simulink library "threeTetherThreeSurfaceCtrl_cl"  (R2022a)
settings: Solver=VariableStepAuto  StartTime=0.0  StopTime=10.0  RelTol=1e-3
undefined symbols (not defined in the file or in its folder): altitudeCtrlShutOffDelay, expOffset, filteredPIDController, filteredPIDController_ul, FLIGHTCONTROLLER, fltCtrl, initialDelay, initializeBussesFromBlock
settings Model: Creator=mcobb  LastModifiedBy=lhill8
settings SolverCC: AlgebraicLoopSolver=TrustRegion
settings DebuggingCC: UnconnectedInputMsg=warning  UnconnectedOutputMsg=warning  UnconnectedLineMsg=warning  SFMachineParentedDataDiag=warning  ArithmeticOperatorsInVariantConditions=warning
settings SFSimCC: CustomCodeUndefinedFunction=UseInterfaceOnly

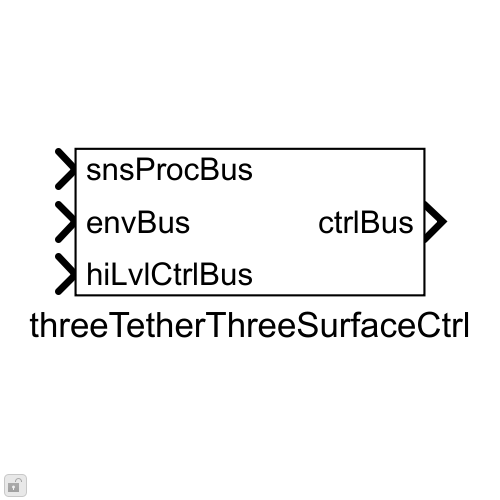
[thumbnail: Simulink's stored preview of the top-level diagram]
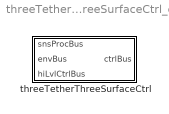
== system threeTetherThreeSurfaceCtrl_cl ==
  threeTetherThreeSurfaceCtrl : Subsystem  LoadFcn=initializeBussesFromBlock(gcb)  InitFcn=initializeBussesFromBlock(gcb)  StartFcn=initializeBussesFromBlock(gcb)  VariantControl=strcmpi(FLIGHTCONTROLLER,'threeTetherThreeSurfaceCtrl')  mask{ctrl=fltCtrl}
      mask prompts: ctrl "Controller Object"

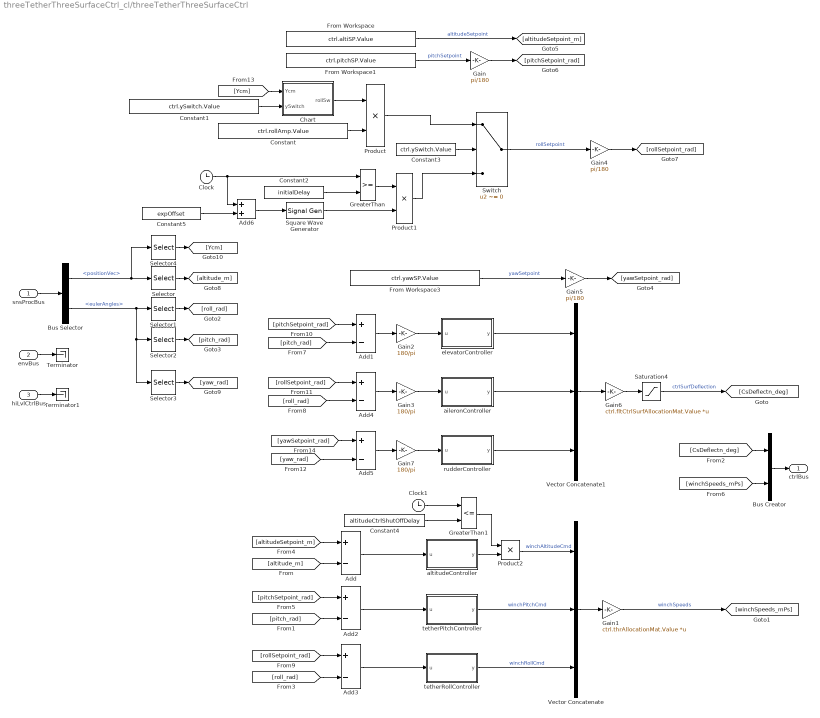
== system threeTetherThreeSurfaceCtrl_cl/threeTetherThreeSurfaceCtrl ==
  snsProcBus : Inport  OutDataTypeStr=Bus: sensorsProcessingBus
  envBus : Inport  Port=2  OutDataTypeStr=Bus: envBus
  hiLvlCtrlBus : Inport  Port=3  OutDataTypeStr=Bus: hiLvlCtrlBus
  Add{,1..5} (6 alike) : Sum  Inputs=+-
  Add6 : Sum
  Bus Creator : BusCreator  Inputs=2  OutDataTypeStr=Bus: fltCtrlBus
  Bus Selector : BusSelector  OutputSignals=positionVec,eulerAngles
  Chart : Stateflow chart  TreatAsAtomicUnit=on
  Clock : Clock
  Clock1 : Clock
  Constant : Constant  Value=ctrl.rollAmp.Value
  Constant1 : Constant  Value=ctrl.ySwitch.Value
  Constant2 : Constant  Value=initialDelay
  Constant3 : Constant  Value=ctrl.ySwitch.Value
  Constant4 : Constant  Value=altitudeCtrlShutOffDelay
  Constant5 : Constant  Value=expOffset
  From Workspace : FromWorkspace  VariableName=ctrl.altiSP.Value
  From Workspace1 : FromWorkspace  VariableName=ctrl.pitchSP.Value
  From Workspace3 : FromWorkspace  VariableName=ctrl.yawSP.Value
  Gain : Gain  Gain=pi/180
  Gain1 : Gain  Gain=ctrl.thrAllocationMat.Value  Multiplication=Matrix(K*u)
  Gain2 : Gain  Gain=180/pi
  Gain3 : Gain  Gain=180/pi
  Gain4 : Gain  Gain=pi/180
  Gain5 : Gain  Gain=pi/180
  Gain6 : Gain  Gain=ctrl.fltCtrlSurfAllocationMat.Value  Multiplication=Matrix(K*u)
  Gain7 : Gain  Gain=180/pi
  GreaterThan : RelationalOperator  OutDataTypeStr=boolean  RndMeth=Simplest  InputSameDT=off
  GreaterThan1 : RelationalOperator  Operator=<=  OutDataTypeStr=boolean  RndMeth=Simplest  InputSameDT=off
  Product : Product
  Product1 : Product
  Product2 : Product
  Saturation4 : Saturate  UpperLimit=ctrl.outputSat.upperLimit.Value  LowerLimit=ctrl.outputSat.lowerLimit.Value
  Selector : Selector  InputPortWidth=3  IndexOptions=Index vector (dialog)  Indices=3  OutputSizes=1
  Selector1 : Selector  InputPortWidth=3  IndexOptions=Index vector (dialog)  Indices=1  OutputSizes=1
  Selector2 : Selector  InputPortWidth=3  IndexOptions=Index vector (dialog)  Indices=2  OutputSizes=1
  Selector3 : Selector  InputPortWidth=3  IndexOptions=Index vector (dialog)  Indices=3  OutputSizes=1
  Selector4 : Selector  InputPortWidth=3  IndexOptions=Index vector (dialog)  Indices=2  OutputSizes=1
  Square Wave Generator : SignalGenerator  WaveForm=square  TimeSource=Use external signal  Amplitude=ctrl.rollAmp.Value  Frequency=1/ctrl.rollPeriod.Value
  Switch : Switch  Criteria=u2 ~= 0  SaturateOnIntegerOverflow=off  InputSameDT=off
  Terminator : Terminator
  Terminator1 : Terminator
  Vector Concatenate : Concatenate  NumInputs=3
  Vector Concatenate1 : Concatenate  NumInputs=3
  aileronController : Subsystem  AncestorBlock=filteredPIDController_ul/filteredPIDController  mask{kp=ctrl.ailerons.kp.Value, ki=ctrl.ailerons.ki.Value, kd=ctrl.ailerons.kd.Value, Value=ctrl.ailerons.tau.Value, externalReset=none}
      mask prompts: kp "Proportional Gain, kp"; ki "Integral Gain, ki"; kd "Derivative Gain, kd"; Value "Time Constant, s"; externalReset "External reset:"
      mask init:
      | initfcn
      mask TypeOptions kp: kp/Gain
      mask TypeOptions ki: ki/Gain
      mask TypeOptions kd: kd/Gain
      mask TypeOptions Value: tau/Value
      mask TypeOptions externalReset: none | rising | falling | either | level | level hold
  altitudeController : Subsystem  AncestorBlock=filteredPIDController_ul/filteredPIDController  mask{kp=ctrl.tetherAlti.kp.Value, ki=ctrl.tetherAlti.ki.Value, kd=ctrl.tetherAlti.kd.Value, Value=ctrl.tetherAlti.tau.Value, externalReset=none}
      mask prompts: kp "Proportional Gain, kp"; ki "Integral Gain, ki"; kd "Derivative Gain, kd"; Value "Time Constant, s"; externalReset "External reset:"
      mask init:
      | initfcn
      mask TypeOptions kp: kp/Gain
      mask TypeOptions ki: ki/Gain
      mask TypeOptions kd: kd/Gain
      mask TypeOptions Value: tau/Value
      mask TypeOptions externalReset: none | rising | falling | either | level | level hold
  elevatorController : Subsystem  AncestorBlock=filteredPIDController_ul/filteredPIDController  mask{kp=ctrl.elevators.kp.Value, ki=ctrl.elevators.ki.Value, kd=ctrl.elevators.kd.Value, Value=ctrl.elevators.tau.Value, externalReset=none}
      mask prompts: kp "Proportional Gain, kp"; ki "Integral Gain, ki"; kd "Derivative Gain, kd"; Value "Time Constant, s"; externalReset "External reset:"
      mask init:
      | initfcn
      mask TypeOptions kp: kp/Gain
      mask TypeOptions ki: ki/Gain
      mask TypeOptions kd: kd/Gain
      mask TypeOptions Value: tau/Value
      mask TypeOptions externalReset: none | rising | falling | either | level | level hold
  rudderController : Subsystem  AncestorBlock=filteredPIDController_ul/filteredPIDController  mask{kp=ctrl.rudder.kp.Value, ki=ctrl.rudder.ki.Value, kd=ctrl.rudder.kd.Value, Value=ctrl.rudder.tau.Value, externalReset=none}
      mask prompts: kp "Proportional Gain, kp"; ki "Integral Gain, ki"; kd "Derivative Gain, kd"; Value "Time Constant, s"; externalReset "External reset:"
      mask init:
      | initfcn
      mask TypeOptions kp: kp/Gain
      mask TypeOptions ki: ki/Gain
      mask TypeOptions kd: kd/Gain
      mask TypeOptions Value: tau/Value
      mask TypeOptions externalReset: none | rising | falling | either | level | level hold
  tetherPitchController : Subsystem  AncestorBlock=filteredPIDController_ul/filteredPIDController  mask{kp=ctrl.tetherPitch.kp.Value, ki=ctrl.tetherPitch.ki.Value, kd=ctrl.tetherPitch.kd.Value, Value=ctrl.tetherPitch.tau.Value, externalReset=none}
      mask prompts: kp "Proportional Gain, kp"; ki "Integral Gain, ki"; kd "Derivative Gain, kd"; Value "Time Constant, s"; externalReset "External reset:"
      mask init:
      | initfcn
      mask TypeOptions kp: kp/Gain
      mask TypeOptions ki: ki/Gain
      mask TypeOptions kd: kd/Gain
      mask TypeOptions Value: tau/Value
      mask TypeOptions externalReset: none | rising | falling | either | level | level hold
  tetherRollController : Subsystem  AncestorBlock=filteredPIDController_ul/filteredPIDController  mask{kp=ctrl.tetherRoll.kp.Value, ki=ctrl.tetherRoll.ki.Value, kd=ctrl.tetherRoll.kd.Value, Value=ctrl.tetherRoll.tau.Value, externalReset=none}
      mask prompts: kp "Proportional Gain, kp"; ki "Integral Gain, ki"; kd "Derivative Gain, kd"; Value "Time Constant, s"; externalReset "External reset:"
      mask init:
      | initfcn
      mask TypeOptions kp: kp/Gain
      mask TypeOptions ki: ki/Gain
      mask TypeOptions kd: kd/Gain
      mask TypeOptions Value: tau/Value
      mask TypeOptions externalReset: none | rising | falling | either | level | level hold
  ctrlBus : Outport  OutDataTypeStr=Bus: fltCtrlBus  VectorParamsAs1DForOutWhenUnconnected=off
  wires:
  Constant5/1 -> Add6/2
  Add6/1 -> Square Wave Generator/1
  Product1/1 -> Switch/3
  altitudeController/1(y) -> Product2/2
  Clock1/1 -> GreaterThan1/1
  Constant4/1 -> GreaterThan1/2
  GreaterThan1/1 -> Product2/1
  Switch/1 -> Gain4/1  "rollSetpoint"
  Constant3/1 -> Switch/2
  Square Wave Generator/1 -> Product1/2
  GreaterThan/1 -> Product1/1
  Constant2/1 -> GreaterThan/2
  Clock/1 -> GreaterThan/1, Add6/1
  hiLvlCtrlBus/1 -> Terminator1/1
  Constant1/1 -> Chart/2(ySwitch)
  Chart/1(rollSw) -> Product/1
  Constant/1 -> Product/2
  [Ycm] -> Chart/1(Ycm)
  Selector4/1 -> [Ycm]
  Selector3/1 -> [yaw_rad]
  rudderController/1(y) -> Vector Concatenate1/3
  Gain7/1 -> rudderController/1(u)
  [yawSetpoint_rad] -> Add5/1
  Add5/1 -> Gain7/1
  [yaw_rad] -> Add5/2
  Gain5/1 -> [yawSetpoint_rad]
  From Workspace3/1 -> Gain5/1  "yawSetpoint"
  Product/1 -> Switch/1
  From Workspace1/1 -> Gain/1  "pitchSetpoint"
  From Workspace/1 -> [altitudeSetpoint_m]  "altitudeSetpoint"
  Selector2/1 -> [pitch_rad]
  Selector1/1 -> [roll_rad]
  Bus Selector/2 -> Selector1/1, Selector2/1, Selector3/1  "<eulerAngles>"
  Bus Selector/1 -> Selector/1, Selector4/1  "<positionVec>"
  [rollSetpoint_rad] -> Add4/1
  [pitchSetpoint_rad] -> Add1/1
  Selector/1 -> [altitude_m]
  Gain4/1 -> [rollSetpoint_rad]
  Gain/1 -> [pitchSetpoint_rad]
  snsProcBus/1 -> Bus Selector/1
  envBus/1 -> Terminator/1
  [winchSpeeds_mPs] -> Bus Creator/2
  [CsDeflectn_deg] -> Bus Creator/1
  Gain1/1 -> [winchSpeeds_mPs]  "winchSpeeds"
  Bus Creator/1 -> ctrlBus/1
  Add1/1 -> Gain2/1
  Gain3/1 -> aileronController/1(u)
  Gain2/1 -> elevatorController/1(u)
  Gain6/1 -> Saturation4/1
  [pitch_rad] -> Add1/2
  Add4/1 -> Gain3/1
  [roll_rad] -> Add4/2
  elevatorController/1(y) -> Vector Concatenate1/1
  aileronController/1(y) -> Vector Concatenate1/2
  Vector Concatenate1/1 -> Gain6/1
  Saturation4/1 -> [CsDeflectn_deg]  "ctrlSurfDeflection"
  Product2/1 -> Vector Concatenate/1  "winchAltitudeCmd"
  tetherPitchController/1(y) -> Vector Concatenate/2  "winchPitchCmd"
  [altitudeSetpoint_m] -> Add/1
  [altitude_m] -> Add/2
  tetherRollController/1(y) -> Vector Concatenate/3  "winchRollCmd"
  [rollSetpoint_rad] -> Add3/1
  [roll_rad] -> Add3/2
  [pitch_rad] -> Add2/2
  [pitchSetpoint_rad] -> Add2/1
  Add/1 -> altitudeController/1(u)
  Add3/1 -> tetherRollController/1(u)
  Add2/1 -> tetherPitchController/1(u)
  Vector Concatenate/1 -> Gain1/1

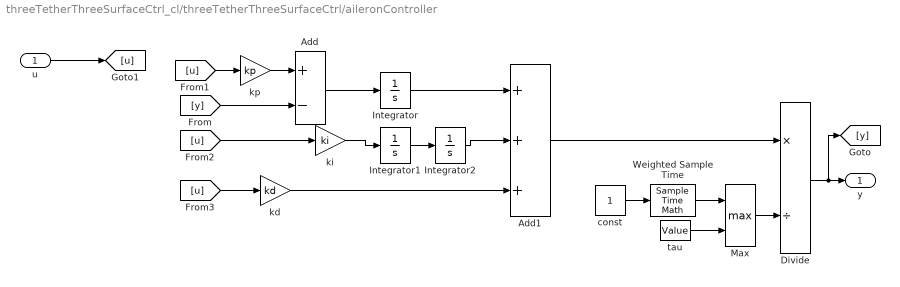
== system threeTetherThreeSurfaceCtrl_cl/threeTetherThreeSurfaceCtrl/aileronController ==
  u : Inport  PortDimensions=1
  Add : Sum  Inputs=+-
  Add1 : Sum  Inputs=+++
  Divide : Product  Inputs=*/
  Integrator : Integrator
  Integrator1 : Integrator
  Integrator2 : Integrator
  Max : MinMax  Function=max  Inputs=2
  Weighted Sample Time : SampleTimeMath  TsampMathOp=Ts Only
  const : Constant
  kd : Gain  Gain=kd
  ki : Gain  Gain=ki
  kp : Gain  Gain=kp
  tau : Constant  Value=Value
  y : Outport  PortDimensions=1  VectorParamsAs1DForOutWhenUnconnected=off
  wires:
  u/1 -> [u]
  kp/1 -> Add/1
  [y] -> Add/2
  Add/1 -> Integrator/1
  [u] -> kp/1
  Max/1 -> Divide/2
  tau/1 -> Max/2
  Integrator1/1 -> Integrator2/1
  ki/1 -> Integrator1/1
  [u] -> ki/1
  [u] -> kd/1
  Integrator2/1 -> Add1/2
  Integrator/1 -> Add1/1
  kd/1 -> Add1/3
  Add1/1 -> Divide/1
  Divide/1 -> [y], y/1
  Weighted Sample Time/1 -> Max/1
  const/1 -> Weighted Sample Time/1

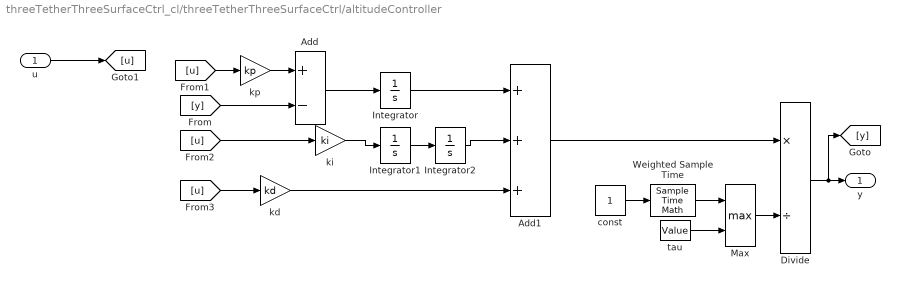
== system threeTetherThreeSurfaceCtrl_cl/threeTetherThreeSurfaceCtrl/altitudeController ==
  u : Inport  PortDimensions=1
  Add : Sum  Inputs=+-
  Add1 : Sum  Inputs=+++
  Divide : Product  Inputs=*/
  Integrator : Integrator
  Integrator1 : Integrator
  Integrator2 : Integrator
  Max : MinMax  Function=max  Inputs=2
  Weighted Sample Time : SampleTimeMath  TsampMathOp=Ts Only
  const : Constant
  kd : Gain  Gain=kd
  ki : Gain  Gain=ki
  kp : Gain  Gain=kp
  tau : Constant  Value=Value
  y : Outport  PortDimensions=1  VectorParamsAs1DForOutWhenUnconnected=off
  wires:
  u/1 -> [u]
  kp/1 -> Add/1
  [y] -> Add/2
  Add/1 -> Integrator/1
  [u] -> kp/1
  Max/1 -> Divide/2
  tau/1 -> Max/2
  Integrator1/1 -> Integrator2/1
  ki/1 -> Integrator1/1
  [u] -> ki/1
  [u] -> kd/1
  Integrator2/1 -> Add1/2
  Integrator/1 -> Add1/1
  kd/1 -> Add1/3
  Add1/1 -> Divide/1
  Divide/1 -> [y], y/1
  Weighted Sample Time/1 -> Max/1
  const/1 -> Weighted Sample Time/1

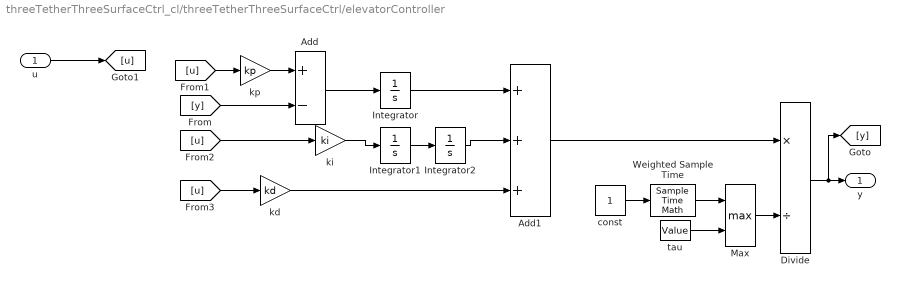
== system threeTetherThreeSurfaceCtrl_cl/threeTetherThreeSurfaceCtrl/elevatorController ==
  u : Inport  PortDimensions=1
  Add : Sum  Inputs=+-
  Add1 : Sum  Inputs=+++
  Divide : Product  Inputs=*/
  Integrator : Integrator
  Integrator1 : Integrator
  Integrator2 : Integrator
  Max : MinMax  Function=max  Inputs=2
  Weighted Sample Time : SampleTimeMath  TsampMathOp=Ts Only
  const : Constant
  kd : Gain  Gain=kd
  ki : Gain  Gain=ki
  kp : Gain  Gain=kp
  tau : Constant  Value=Value
  y : Outport  PortDimensions=1  VectorParamsAs1DForOutWhenUnconnected=off
  wires:
  u/1 -> [u]
  kp/1 -> Add/1
  [y] -> Add/2
  Add/1 -> Integrator/1
  [u] -> kp/1
  Max/1 -> Divide/2
  tau/1 -> Max/2
  Integrator1/1 -> Integrator2/1
  ki/1 -> Integrator1/1
  [u] -> ki/1
  [u] -> kd/1
  Integrator2/1 -> Add1/2
  Integrator/1 -> Add1/1
  kd/1 -> Add1/3
  Add1/1 -> Divide/1
  Divide/1 -> [y], y/1
  Weighted Sample Time/1 -> Max/1
  const/1 -> Weighted Sample Time/1

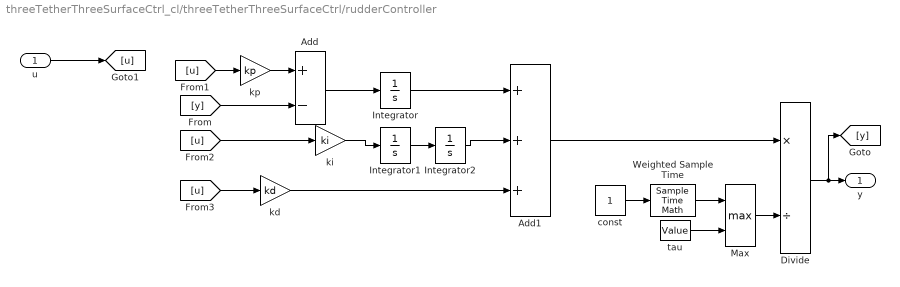
== system threeTetherThreeSurfaceCtrl_cl/threeTetherThreeSurfaceCtrl/rudderController ==
  u : Inport  PortDimensions=1
  Add : Sum  Inputs=+-
  Add1 : Sum  Inputs=+++
  Divide : Product  Inputs=*/
  Integrator : Integrator
  Integrator1 : Integrator
  Integrator2 : Integrator
  Max : MinMax  Function=max  Inputs=2
  Weighted Sample Time : SampleTimeMath  TsampMathOp=Ts Only
  const : Constant
  kd : Gain  Gain=kd
  ki : Gain  Gain=ki
  kp : Gain  Gain=kp
  tau : Constant  Value=Value
  y : Outport  PortDimensions=1  VectorParamsAs1DForOutWhenUnconnected=off
  wires:
  u/1 -> [u]
  kp/1 -> Add/1
  [y] -> Add/2
  Add/1 -> Integrator/1
  [u] -> kp/1
  Max/1 -> Divide/2
  tau/1 -> Max/2
  Integrator1/1 -> Integrator2/1
  ki/1 -> Integrator1/1
  [u] -> ki/1
  [u] -> kd/1
  Integrator2/1 -> Add1/2
  Integrator/1 -> Add1/1
  kd/1 -> Add1/3
  Add1/1 -> Divide/1
  Divide/1 -> [y], y/1
  Weighted Sample Time/1 -> Max/1
  const/1 -> Weighted Sample Time/1

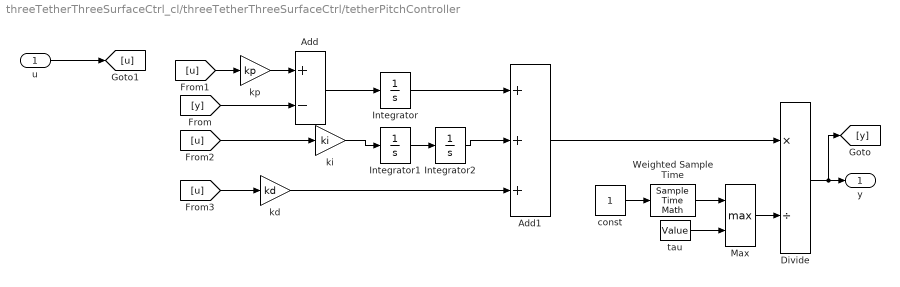
== system threeTetherThreeSurfaceCtrl_cl/threeTetherThreeSurfaceCtrl/tetherPitchController ==
  u : Inport  PortDimensions=1
  Add : Sum  Inputs=+-
  Add1 : Sum  Inputs=+++
  Divide : Product  Inputs=*/
  Integrator : Integrator
  Integrator1 : Integrator
  Integrator2 : Integrator
  Max : MinMax  Function=max  Inputs=2
  Weighted Sample Time : SampleTimeMath  TsampMathOp=Ts Only
  const : Constant
  kd : Gain  Gain=kd
  ki : Gain  Gain=ki
  kp : Gain  Gain=kp
  tau : Constant  Value=Value
  y : Outport  PortDimensions=1  VectorParamsAs1DForOutWhenUnconnected=off
  wires:
  u/1 -> [u]
  kp/1 -> Add/1
  [y] -> Add/2
  Add/1 -> Integrator/1
  [u] -> kp/1
  Max/1 -> Divide/2
  tau/1 -> Max/2
  Integrator1/1 -> Integrator2/1
  ki/1 -> Integrator1/1
  [u] -> ki/1
  [u] -> kd/1
  Integrator2/1 -> Add1/2
  Integrator/1 -> Add1/1
  kd/1 -> Add1/3
  Add1/1 -> Divide/1
  Divide/1 -> [y], y/1
  Weighted Sample Time/1 -> Max/1
  const/1 -> Weighted Sample Time/1

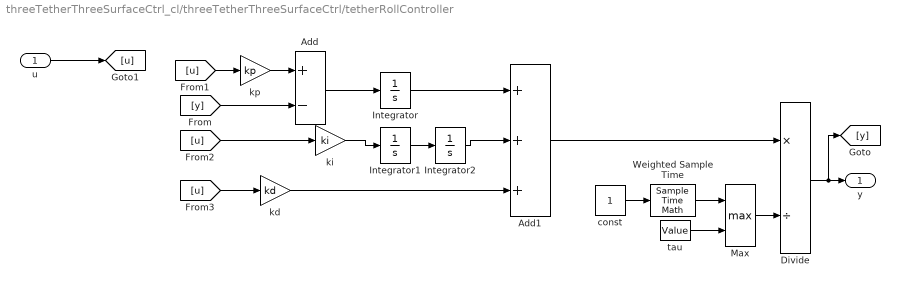
== system threeTetherThreeSurfaceCtrl_cl/threeTetherThreeSurfaceCtrl/tetherRollController ==
  u : Inport  PortDimensions=1
  Add : Sum  Inputs=+-
  Add1 : Sum  Inputs=+++
  Divide : Product  Inputs=*/
  Integrator : Integrator
  Integrator1 : Integrator
  Integrator2 : Integrator
  Max : MinMax  Function=max  Inputs=2
  Weighted Sample Time : SampleTimeMath  TsampMathOp=Ts Only
  const : Constant
  kd : Gain  Gain=kd
  ki : Gain  Gain=ki
  kp : Gain  Gain=kp
  tau : Constant  Value=Value
  y : Outport  PortDimensions=1  VectorParamsAs1DForOutWhenUnconnected=off
  wires:
  u/1 -> [u]
  kp/1 -> Add/1
  [y] -> Add/2
  Add/1 -> Integrator/1
  [u] -> kp/1
  Max/1 -> Divide/2
  tau/1 -> Max/2
  Integrator1/1 -> Integrator2/1
  ki/1 -> Integrator1/1
  [u] -> ki/1
  [u] -> kd/1
  Integrator2/1 -> Add1/2
  Integrator/1 -> Add1/1
  kd/1 -> Add1/3
  Add1/1 -> Divide/1
  Divide/1 -> [y], y/1
  Weighted Sample Time/1 -> Max/1
  const/1 -> Weighted Sample Time/1

== stateflow chart threeTetherThreeSurfaceCtrl_cl/threeTetherThreeSurfaceCtrl/Chart ==
  state PositiveRoll
    entry:
    rollSw = 1;
  state NegativeRoll
    entry:
    rollSw = -1;
  (default) -> PositiveRoll
  NegativeRoll -> PositiveRoll : [Ycm>ySwitch]
  PositiveRoll -> NegativeRoll : [Ycm<-ySwitch]
  data: Ycm input; rollSw output; ySwitch input
